simulink model "testTrajectory"  (R2020a)
settings: Solver=VariableStepAuto  StartTime=0.0  StopTime=10.0  RelTol=1e-3
values from neighbouring files (symbols this model uses):
  gait_time = 1    [Parameters.m]
  step_height = 0.1    [Parameters.m]
  step_time = gait_time/2    (= 0.5)    [Parameters.m]
  Xc_i = 0    [Parameters.m]
libraries: simulink x2
settings Model: Creator=ashut  LastModifiedBy=ashut

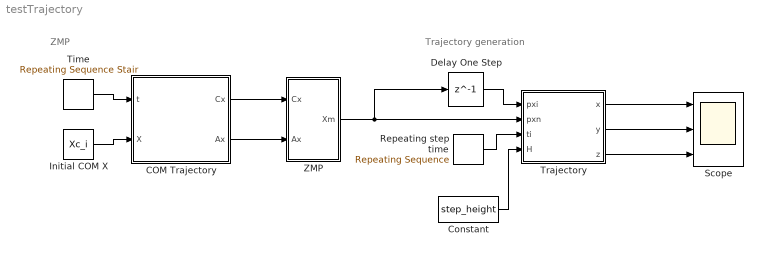
== system testTrajectory ==
  note: Trajectory generation
  note: ZMP
  COM Trajectory : MATLAB Function  TreatAsAtomicUnit=on
  Constant : Constant  Value=step_height
  Delay One Step : Delay  DelayLength=1
  Initial COM X : Constant  Value=Xc_i
  Repeating step time : simulink/Sources/Repeating Sequence  rep_seq_t=[0 step_time]  rep_seq_y=[0 step_time]
  Scope : Scope  NumInputPorts=3
  Time : simulink/Sources/Repeating Sequence Stair  OutValues=[0:gait_time:10].'  tsamp=gait_time  OutMin=[]  OutMax=[]  OutDataTypeStr=double  OutputDataTypeScalingMode=double  OutDataType=fixdt(0,8)  ConRadixGroup=Best Precision: Vector-wise  OutScaling=2^-12
  Trajectory : MATLAB Function  TreatAsAtomicUnit=on
  ZMP : MATLAB Function  TreatAsAtomicUnit=on
  wires:
  Initial COM X/1 -> COM Trajectory/2(X)
  Trajectory/3(z) -> Scope/3
  Trajectory/2(y) -> Scope/2
  Constant/1 -> Trajectory/4(H)
  Delay One Step/1 -> Trajectory/1(pxi)
  Trajectory/1(x) -> Scope/1
  ZMP/1(Xm) -> Delay One Step/1, Trajectory/2(pxn)
  COM Trajectory/1(Cx) -> ZMP/1(Cx)
  COM Trajectory/2(Ax) -> ZMP/2(Ax)
  Repeating step time/1 -> Trajectory/3(ti)
  Time/1 -> COM Trajectory/1(t)

== matlab function testTrajectory/Trajectory ==
  data: x output; y output; pxi input; z output; pxn input; ti input; H input
function[x,y,z] = Trajectory(pxi,pxn,ti,H)
% pxi is cuttrent x position of endpoint
% pxn is final x position of enpoint
% ti is the real time
% H is the height of the step

% These all are in world frame
step_time = 0.5;
x = pxi + sin((pi/2*step_time)*ti)*abs(pxn-pxi);
y = 0;
z = sin((pi/step_time)*ti)*(H);

== matlab function testTrajectory/ZMP ==
  data: Cx input; Ax input; Xm output
function Xm  = ZMP(Cx,Ax)

% g and h defined in Parameters.m
% h here is COM height(z-cordinate) from world/path
h = 0.25;
g = 9.8066;
Xm = Cx - (h/g)*(Ax);

== matlab function testTrajectory/COM Trajectory ==
  data: t input; Cx output; X input; Ax output
function[Cx,Ax] = COM_Trajectory(t,X)
% Here t is sample time
Cx = 0.1*t^2 + X ;
% Vx = 0.2*t;
Ax = 0.2;
